simulink model "model_1mode"  (R2020a)
settings: Solver=VariableStepAuto  StartTime=0.0  StopTime=Inf  RelTol=1e-3
libraries: dspobslib x1
settings Model: Creator=Dinh-Viet-Toan  LastModifiedBy=Dinh-Viet-Toan

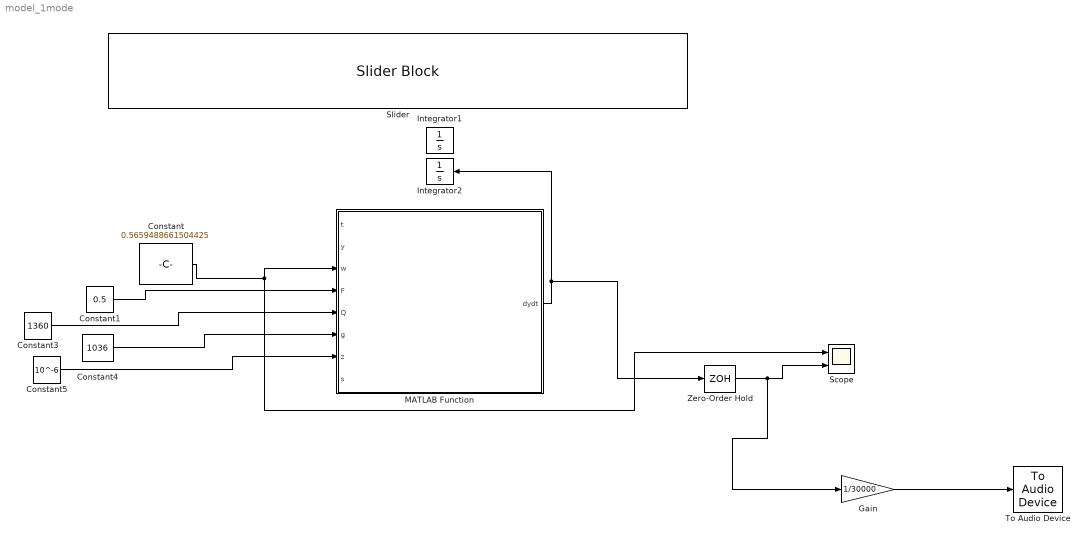
== system model_1mode ==
  Constant : Constant  Value=0.5659488661504425
  Constant1 : Constant  Value=0.5
  Constant3 : Constant  Value=1360
  Constant4 : Constant  Value=1036
  Constant5 : Constant  Value=10^-6
  Gain : Gain  Gain=1/30000
  Integrator1 : Integrator
  Integrator2 : Integrator  InitialCondition=0.01
  MATLAB Function : MATLAB Function  TreatAsAtomicUnit=on
  Scope : Scope  NumInputPorts=2
  Slider : SliderBlock  ScaleMin=0.001  ScaleMax=1
  To Audio Device : dspobslib/To Audio Device  deviceName=Default  inheritSampleRate=off  sampleRate=44100  deviceDatatype=Determine from input data type  autoBufferSize=on  bufferSize=4096  queueDuration=1.0  defaultOutputChannelMapping=on  outputChannelMapping=1:2  outputNumUnderrunSamples=off
      settings: SourceProductBaseCode=DS
  Zero-Order Hold : ZeroOrderHold  SampleTime=1/22050
  wires:
  Constant/1 -> Scope/1, MATLAB Function/3(w)
  Constant3/1 -> MATLAB Function/5(Q)
  Constant4/1 -> MATLAB Function/6(g)
  Constant5/1 -> MATLAB Function/7(z)
  Constant1/1 -> MATLAB Function/4(F)
  MATLAB Function/1(dydt) -> Integrator2/1, Zero-Order Hold/1
  Zero-Order Hold/1 -> Gain/1, Scope/2
  Gain/1 -> To Audio Device/1

== matlab function model_1mode/MATLAB Function ==
  data: t input; dydt output; y input; w input; F input; Q input; g input; z input; s input
function dydt = systdyn_1mode(t,y,w,F,Q,g,z,s)
dudt = (z*y(2)*(g - y(1)))/(s + (g - y(1))^2)^(1/4) - (z*y(2)*(y(1) - g + 1))/(s + (g - y(1))^2)^(1/4) + (z*y(2)*(g - y(1))^2*(y(1) - g + 1))/(2*(s + (g - y(1))^2)^(5/4));

% Ecriture vectorielle Y'=F(Y)
dydt = [y(2); -(w/Q)*y(2) - w^2*y(1) + F*dudt];
end
